simulink model "MyTransmCU_RTW"  (Simulink 10.3)
settings: Solver=ode1  StartTime=0.0  StopTime=inf  FixedStep=0.0002  RelTol=1e-3
PreLoadFcn:
  | vehicle = 'Car'; if ~length(which('cmself')), cmenv; end
  | MyTransmCU_RTW_bus
InitFcn:
  | vehicle = 'Car'; if ~length(which('cmself')), cmenv; end
  | MyTransmCU_RTW_bus
libraries: simulink x2, CarMaker4SL x1
Description:
  | CarMaker Plug-in Model Target
settings Model: Creator=IPG  LastModifiedBy=IPG  MultithreadedSim=on
settings DataIOCC: SaveFormat=Dataset  SignalLoggingSaveFormat=Dataset  ReturnWorkspaceOutputs=on
settings OptimizationCC: ExpressionDepthLimit=128  LifeSpan=auto
settings DebuggingCC: UnderspecifiedInitializationDetection=Simplified  MergeDetectMultiDrivingBlocksExec=error  FcnCallInpInsideContextMsg=error  StateNameClashWarn=none  SFUnexpectedBacktrackingDiag=error  SFNoUnconditionalDefaultTransitionDiag=error  SFExecutionAtInitializationDiag=warning  ArithmeticOperatorsInVariantConditions=error
settings HardwareCC: ProdBitPerPointer=64  ProdBitPerSizeT=64  ProdBitPerPtrDiffT=64  ProdLargestAtomicFloat=Float  ProdIntDivRoundTo=Zero  ProdEndianess=LittleEndian  ProdWordSize=64  ProdHWDeviceType=Intel->x86-64 (Windows64)
settings ModelReferenceCC: PropagateSignalLabelsOutOfModel=on
settings SFSimCC: SimUseLocalCustomCode=on  CustomCodeUndefinedFunction=FilterOut
settings RTWCC: Description=CarMaker Plug-in Model Target  SystemTargetFile=CarMaker.tlc  TemplateMakefile=CarMaker_unix-linux64.tmf  RTWUseLocalCustomCode=on
settings CodeAppCC: MaxIdLength=127  StateflowObjectComments=off
settings STFCustomTargetCC: TargetLangStandard=C99 (ISO)  CombineOutputUpdateFcns=on  MatFileLogging=on  CodeInterfacePackaging=Reusable function  GRTInterface=off  GenerateAllocFcn=on  SystemTargetFile=CarMaker.tlc
settings GRTTargetCC: TargetLangStandard=C99 (ISO)  ParMdlRefBuildCompliant=off  CompOptLevelCompliant=off  ConcurrentExecutionCompliant=off  CombineOutputUpdateFcns=on  CodeInterfacePackaging=Reusable function  CPPClassGenCompliant=off  GRTInterface=off  GenerateAllocFcn=on  UseToolchainInfoCompliant=off
settings CustomProperty: DataType=string
settings EnumStrPairs: String=Car
settings ConfigComp: CovMetricSettings=dwe  CovSaveCumulativeToWorkspaceVar=off  CovSaveSingleToWorkspaceVar=off  CovExternalEMLEnable=on

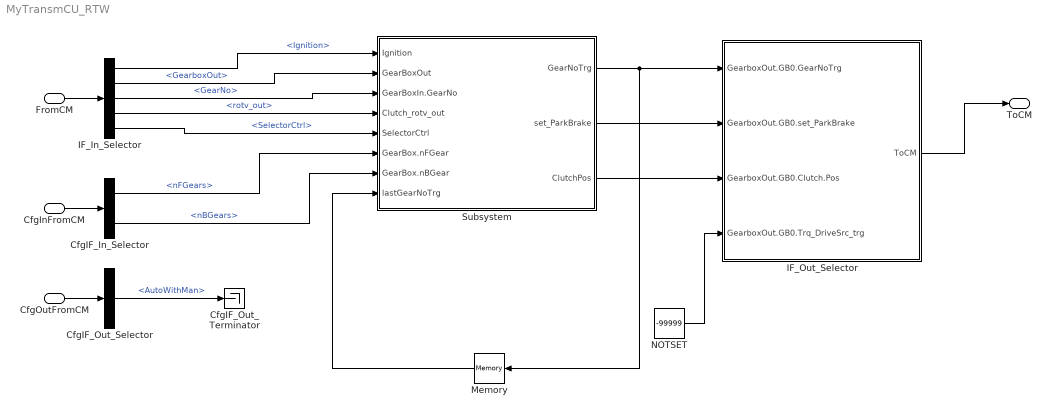
== system MyTransmCU_RTW ==
  FromCM : Inport  OutDataTypeStr=Bus: cmPTTransmCUIn
  CfgInFromCM : Inport  Port=2  OutDataTypeStr=Bus: cmPTTransmCUCfgIn
  CfgOutFromCM : Inport  Port=3  OutDataTypeStr=Bus: cmPTTransmCUCfgOut
  CfgIF_In_Selector : BusSelector  OutputSignals=Gearbox.GB0.nFGears,Gearbox.GB0.nBGears
  CfgIF_Out_Selector : BusSelector  OutputSignals=AutoWithMan
  CfgIF_Out_Terminator : Terminator
  IF_In_Selector : BusSelector  OutputSignals=Ignition,GearboxOut,GearboxIn.GB0.GearNo,GearboxIn.GB0.rotv_out,SelectorCtrl
  IF_Out_Selector : Subsystem  mask(Signal Selection){}
      mask help: Signal Selection Block
      settings: OpenFcn=cmSignalSelect('SignalSelection_CB',gcb)
  Memory : Memory
  NOTSET : Constant  Value=-99999
  Subsystem : Subsystem
  ToCM : Outport  OutDataTypeStr=Bus: cmPTTransmCUOut
  wires:
  FromCM/1 -> IF_In_Selector/1
  IF_Out_Selector/1(ToCM) -> ToCM/1
  CfgInFromCM/1 -> CfgIF_In_Selector/1
  CfgIF_In_Selector/1 -> Subsystem/6(GearBox.nFGear)  "<nFGears>"
  CfgOutFromCM/1 -> CfgIF_Out_Selector/1
  CfgIF_Out_Selector/1 -> CfgIF_Out_Terminator/1  "<AutoWithMan>"
  Memory/1 -> Subsystem/8(lastGearNoTrg)
  Subsystem/2(set_ParkBrake) -> IF_Out_Selector/2(GearboxOut.GB0.set_ParkBrake)
  IF_In_Selector/3 -> Subsystem/3(GearBoxIn.GearNo)  "<GearNo>"
  IF_In_Selector/5 -> Subsystem/5(SelectorCtrl)  "<SelectorCtrl>"
  Subsystem/3(ClutchPos) -> IF_Out_Selector/3(GearboxOut.GB0.Clutch.Pos)
  Subsystem/1(GearNoTrg) -> Memory/1, IF_Out_Selector/1(GearboxOut.GB0.GearNoTrg)
  NOTSET/1 -> IF_Out_Selector/4(GearboxOut.GB0.Trq_DriveSrc_trg)
  IF_In_Selector/4 -> Subsystem/4(Clutch_rotv_out)  "<rotv_out>"
  CfgIF_In_Selector/2 -> Subsystem/7(GearBox.nBGear)  "<nBGears>"
  IF_In_Selector/1 -> Subsystem/1(Ignition)  "<Ignition>"
  IF_In_Selector/2 -> Subsystem/2(GearBoxOut)  "<GearboxOut>"

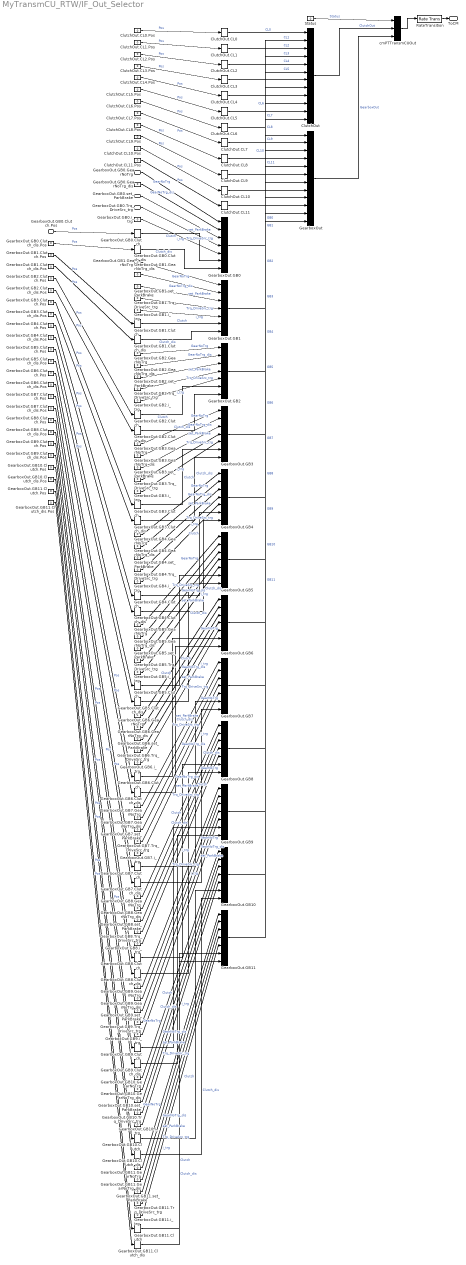
== system MyTransmCU_RTW/IF_Out_Selector ==
  GearboxOut.GB0.GearNoTrg : Inport
  GearboxOut.GB0.set_ParkBrake : Inport  Port=2
  GearboxOut.GB0.Clutch.Pos : Inport  Port=3
  GearboxOut.GB0.Trq_DriveSrc_trg : Inport  Port=4
  ClutchOut : BusCreator  Inputs=12
  ClutchOut.CL{0..11} (12 alike) : BusCreator  Inputs=1
  ClutchOut.CL0.Pos : Constant  Value=0
  ClutchOut.CL1.Pos : Constant  Value=0
  ClutchOut.CL10.Pos : Constant  Value=0
  ClutchOut.CL11.Pos : Constant  Value=0
  ClutchOut.CL2.Pos : Constant  Value=0
  ClutchOut.CL3.Pos : Constant  Value=0
  ClutchOut.CL4.Pos : Constant  Value=0
  ClutchOut.CL5.Pos : Constant  Value=0
  ClutchOut.CL6.Pos : Constant  Value=0
  ClutchOut.CL7.Pos : Constant  Value=0
  ClutchOut.CL8.Pos : Constant  Value=0
  ClutchOut.CL9.Pos : Constant  Value=0
  GearboxOut : BusCreator  Inputs=12
  GearboxOut.GB{0..11} (12 alike) : BusCreator  Inputs=7
  GearboxOut.GB0.Clutch : BusCreator  Inputs=1
  GearboxOut.GB0.Clutch_dis : BusCreator  Inputs=1
  GearboxOut.GB0.Clutch_dis.Pos : Constant  Value=0
  GearboxOut.GB0.GearNoTrg_dis : Constant  Value=0
  GearboxOut.GB0.i_trg : Constant  Value=0
  GearboxOut.GB1.Clutch : BusCreator  Inputs=1
  GearboxOut.GB1.Clutch.Pos : Constant  Value=0
  GearboxOut.GB1.Clutch_dis : BusCreator  Inputs=1
  GearboxOut.GB1.Clutch_dis.Pos : Constant  Value=0
  GearboxOut.GB1.GearNoTrg : Constant  Value=0
  GearboxOut.GB1.GearNoTrg_dis : Constant  Value=0
  GearboxOut.GB1.Trq_DriveSrc_trg : Constant  Value=0
  GearboxOut.GB1.i_trg : Constant  Value=0
  GearboxOut.GB1.set_ParkBrake : Constant  Value=0
  GearboxOut.GB10.Clutch : BusCreator  Inputs=1
  GearboxOut.GB10.Clutch.Pos : Constant  Value=0
  GearboxOut.GB10.Clutch_dis : BusCreator  Inputs=1
  GearboxOut.GB10.Clutch_dis.Pos : Constant  Value=0
  GearboxOut.GB10.GearNoTrg : Constant  Value=0
  GearboxOut.GB10.GearNoTrg_dis : Constant  Value=0
  GearboxOut.GB10.Trq_DriveSrc_trg : Constant  Value=0
  GearboxOut.GB10.i_trg : Constant  Value=0
  GearboxOut.GB10.set_ParkBrake : Constant  Value=0
  GearboxOut.GB11.Clutch : BusCreator  Inputs=1
  GearboxOut.GB11.Clutch.Pos : Constant  Value=0
  GearboxOut.GB11.Clutch_dis : BusCreator  Inputs=1
  GearboxOut.GB11.Clutch_dis.Pos : Constant  Value=0
  GearboxOut.GB11.GearNoTrg : Constant  Value=0
  GearboxOut.GB11.GearNoTrg_dis : Constant  Value=0
  GearboxOut.GB11.Trq_DriveSrc_trg : Constant  Value=0
  GearboxOut.GB11.i_trg : Constant  Value=0
  GearboxOut.GB11.set_ParkBrake : Constant  Value=0
  GearboxOut.GB2.Clutch : BusCreator  Inputs=1
  GearboxOut.GB2.Clutch.Pos : Constant  Value=0
  GearboxOut.GB2.Clutch_dis : BusCreator  Inputs=1
  GearboxOut.GB2.Clutch_dis.Pos : Constant  Value=0
  GearboxOut.GB2.GearNoTrg : Constant  Value=0
  GearboxOut.GB2.GearNoTrg_dis : Constant  Value=0
  GearboxOut.GB2.Trq_DriveSrc_trg : Constant  Value=0
  GearboxOut.GB2.i_trg : Constant  Value=0
  GearboxOut.GB2.set_ParkBrake : Constant  Value=0
  GearboxOut.GB3.Clutch : BusCreator  Inputs=1
  GearboxOut.GB3.Clutch.Pos : Constant  Value=0
  GearboxOut.GB3.Clutch_dis : BusCreator  Inputs=1
  GearboxOut.GB3.Clutch_dis.Pos : Constant  Value=0
  GearboxOut.GB3.GearNoTrg : Constant  Value=0
  GearboxOut.GB3.GearNoTrg_dis : Constant  Value=0
  GearboxOut.GB3.Trq_DriveSrc_trg : Constant  Value=0
  GearboxOut.GB3.i_trg : Constant  Value=0
  GearboxOut.GB3.set_ParkBrake : Constant  Value=0
  GearboxOut.GB4.Clutch : BusCreator  Inputs=1
  GearboxOut.GB4.Clutch.Pos : Constant  Value=0
  GearboxOut.GB4.Clutch_dis : BusCreator  Inputs=1
  GearboxOut.GB4.Clutch_dis.Pos : Constant  Value=0
  GearboxOut.GB4.GearNoTrg : Constant  Value=0
  GearboxOut.GB4.GearNoTrg_dis : Constant  Value=0
  GearboxOut.GB4.Trq_DriveSrc_trg : Constant  Value=0
  GearboxOut.GB4.i_trg : Constant  Value=0
  GearboxOut.GB4.set_ParkBrake : Constant  Value=0
  GearboxOut.GB5.Clutch : BusCreator  Inputs=1
  GearboxOut.GB5.Clutch.Pos : Constant  Value=0
  GearboxOut.GB5.Clutch_dis : BusCreator  Inputs=1
  GearboxOut.GB5.Clutch_dis.Pos : Constant  Value=0
  GearboxOut.GB5.GearNoTrg : Constant  Value=0
  GearboxOut.GB5.GearNoTrg_dis : Constant  Value=0
  GearboxOut.GB5.Trq_DriveSrc_trg : Constant  Value=0
  GearboxOut.GB5.i_trg : Constant  Value=0
  GearboxOut.GB5.set_ParkBrake : Constant  Value=0
  GearboxOut.GB6.Clutch : BusCreator  Inputs=1
  GearboxOut.GB6.Clutch.Pos : Constant  Value=0
  GearboxOut.GB6.Clutch_dis : BusCreator  Inputs=1
  GearboxOut.GB6.Clutch_dis.Pos : Constant  Value=0
  GearboxOut.GB6.GearNoTrg : Constant  Value=0
  GearboxOut.GB6.GearNoTrg_dis : Constant  Value=0
  GearboxOut.GB6.Trq_DriveSrc_trg : Constant  Value=0
  GearboxOut.GB6.i_trg : Constant  Value=0
  GearboxOut.GB6.set_ParkBrake : Constant  Value=0
  GearboxOut.GB7.Clutch : BusCreator  Inputs=1
  GearboxOut.GB7.Clutch.Pos : Constant  Value=0
  GearboxOut.GB7.Clutch_dis : BusCreator  Inputs=1
  GearboxOut.GB7.Clutch_dis.Pos : Constant  Value=0
  GearboxOut.GB7.GearNoTrg : Constant  Value=0
  GearboxOut.GB7.GearNoTrg_dis : Constant  Value=0
  GearboxOut.GB7.Trq_DriveSrc_trg : Constant  Value=0
  GearboxOut.GB7.i_trg : Constant  Value=0
  GearboxOut.GB7.set_ParkBrake : Constant  Value=0
  GearboxOut.GB8.Clutch : BusCreator  Inputs=1
  GearboxOut.GB8.Clutch.Pos : Constant  Value=0
  GearboxOut.GB8.Clutch_dis : BusCreator  Inputs=1
  GearboxOut.GB8.Clutch_dis.Pos : Constant  Value=0
  GearboxOut.GB8.GearNoTrg : Constant  Value=0
  GearboxOut.GB8.GearNoTrg_dis : Constant  Value=0
  GearboxOut.GB8.Trq_DriveSrc_trg : Constant  Value=0
  GearboxOut.GB8.i_trg : Constant  Value=0
  GearboxOut.GB8.set_ParkBrake : Constant  Value=0
  GearboxOut.GB9.Clutch : BusCreator  Inputs=1
  GearboxOut.GB9.Clutch.Pos : Constant  Value=0
  GearboxOut.GB9.Clutch_dis : BusCreator  Inputs=1
  GearboxOut.GB9.Clutch_dis.Pos : Constant  Value=0
  GearboxOut.GB9.GearNoTrg : Constant  Value=0
  GearboxOut.GB9.GearNoTrg_dis : Constant  Value=0
  GearboxOut.GB9.Trq_DriveSrc_trg : Constant  Value=0
  GearboxOut.GB9.i_trg : Constant  Value=0
  GearboxOut.GB9.set_ParkBrake : Constant  Value=0
  RateTransition : RateTransition  OutPortSampleTime=str2num(get_param(bdroot,'FixedStep'))
  Status : Constant  Value=0
  cmPTTransmCUOut : BusCreator  Inputs=3
  ToCM : Outport
  wires:
  RateTransition/1 -> ToCM/1
  cmPTTransmCUOut/1 -> RateTransition/1
  Status/1 -> cmPTTransmCUOut/1  "Status"
  ClutchOut/1 -> cmPTTransmCUOut/2  "ClutchOut"
  ClutchOut.CL0/1 -> ClutchOut/1  "CL0"
  ClutchOut.CL0.Pos/1 -> ClutchOut.CL0/1  "Pos"
  ClutchOut.CL1/1 -> ClutchOut/2  "CL1"
  ClutchOut.CL1.Pos/1 -> ClutchOut.CL1/1  "Pos"
  ClutchOut.CL2/1 -> ClutchOut/3  "CL2"
  ClutchOut.CL2.Pos/1 -> ClutchOut.CL2/1  "Pos"
  ClutchOut.CL3/1 -> ClutchOut/4  "CL3"
  ClutchOut.CL3.Pos/1 -> ClutchOut.CL3/1  "Pos"
  ClutchOut.CL4/1 -> ClutchOut/5  "CL4"
  ClutchOut.CL4.Pos/1 -> ClutchOut.CL4/1  "Pos"
  ClutchOut.CL5/1 -> ClutchOut/6  "CL5"
  ClutchOut.CL5.Pos/1 -> ClutchOut.CL5/1  "Pos"
  ClutchOut.CL6/1 -> ClutchOut/7  "CL6"
  ClutchOut.CL6.Pos/1 -> ClutchOut.CL6/1  "Pos"
  ClutchOut.CL7/1 -> ClutchOut/8  "CL7"
  ClutchOut.CL7.Pos/1 -> ClutchOut.CL7/1  "Pos"
  ClutchOut.CL8/1 -> ClutchOut/9  "CL8"
  ClutchOut.CL8.Pos/1 -> ClutchOut.CL8/1  "Pos"
  ClutchOut.CL9/1 -> ClutchOut/10  "CL9"
  ClutchOut.CL9.Pos/1 -> ClutchOut.CL9/1  "Pos"
  ClutchOut.CL10/1 -> ClutchOut/11  "CL10"
  ClutchOut.CL10.Pos/1 -> ClutchOut.CL10/1  "Pos"
  ClutchOut.CL11/1 -> ClutchOut/12  "CL11"
  ClutchOut.CL11.Pos/1 -> ClutchOut.CL11/1  "Pos"
  GearboxOut/1 -> cmPTTransmCUOut/3  "GearboxOut"
  GearboxOut.GB0/1 -> GearboxOut/1  "GB0"
  GearboxOut.GB0.GearNoTrg_dis/1 -> GearboxOut.GB0/2  "GearNoTrg_dis"
  GearboxOut.GB0.i_trg/1 -> GearboxOut.GB0/5  "i_trg"
  GearboxOut.GB0.Clutch/1 -> GearboxOut.GB0/6  "Clutch"
  GearboxOut.GB0.Clutch_dis/1 -> GearboxOut.GB0/7  "Clutch_dis"
  GearboxOut.GB0.Clutch_dis.Pos/1 -> GearboxOut.GB0.Clutch_dis/1  "Pos"
  GearboxOut.GB1/1 -> GearboxOut/2  "GB1"
  GearboxOut.GB1.GearNoTrg/1 -> GearboxOut.GB1/1  "GearNoTrg"
  GearboxOut.GB1.GearNoTrg_dis/1 -> GearboxOut.GB1/2  "GearNoTrg_dis"
  GearboxOut.GB1.set_ParkBrake/1 -> GearboxOut.GB1/3  "set_ParkBrake"
  GearboxOut.GB1.Trq_DriveSrc_trg/1 -> GearboxOut.GB1/4  "Trq_DriveSrc_trg"
  GearboxOut.GB1.i_trg/1 -> GearboxOut.GB1/5  "i_trg"
  GearboxOut.GB1.Clutch/1 -> GearboxOut.GB1/6  "Clutch"
  GearboxOut.GB1.Clutch.Pos/1 -> GearboxOut.GB1.Clutch/1  "Pos"
  GearboxOut.GB1.Clutch_dis/1 -> GearboxOut.GB1/7  "Clutch_dis"
  GearboxOut.GB1.Clutch_dis.Pos/1 -> GearboxOut.GB1.Clutch_dis/1  "Pos"
  GearboxOut.GB2/1 -> GearboxOut/3  "GB2"
  GearboxOut.GB2.GearNoTrg/1 -> GearboxOut.GB2/1  "GearNoTrg"
  GearboxOut.GB2.GearNoTrg_dis/1 -> GearboxOut.GB2/2  "GearNoTrg_dis"
  GearboxOut.GB2.set_ParkBrake/1 -> GearboxOut.GB2/3  "set_ParkBrake"
  GearboxOut.GB2.Trq_DriveSrc_trg/1 -> GearboxOut.GB2/4  "Trq_DriveSrc_trg"
  GearboxOut.GB2.i_trg/1 -> GearboxOut.GB2/5  "i_trg"
  GearboxOut.GB2.Clutch/1 -> GearboxOut.GB2/6  "Clutch"
  GearboxOut.GB2.Clutch.Pos/1 -> GearboxOut.GB2.Clutch/1  "Pos"
  GearboxOut.GB2.Clutch_dis/1 -> GearboxOut.GB2/7  "Clutch_dis"
  GearboxOut.GB2.Clutch_dis.Pos/1 -> GearboxOut.GB2.Clutch_dis/1  "Pos"
  GearboxOut.GB3/1 -> GearboxOut/4  "GB3"
  GearboxOut.GB3.GearNoTrg/1 -> GearboxOut.GB3/1  "GearNoTrg"
  GearboxOut.GB3.GearNoTrg_dis/1 -> GearboxOut.GB3/2  "GearNoTrg_dis"
  GearboxOut.GB3.set_ParkBrake/1 -> GearboxOut.GB3/3  "set_ParkBrake"
  GearboxOut.GB3.Trq_DriveSrc_trg/1 -> GearboxOut.GB3/4  "Trq_DriveSrc_trg"
  GearboxOut.GB3.i_trg/1 -> GearboxOut.GB3/5  "i_trg"
  GearboxOut.GB3.Clutch/1 -> GearboxOut.GB3/6  "Clutch"
  GearboxOut.GB3.Clutch.Pos/1 -> GearboxOut.GB3.Clutch/1  "Pos"
  GearboxOut.GB3.Clutch_dis/1 -> GearboxOut.GB3/7  "Clutch_dis"
  GearboxOut.GB3.Clutch_dis.Pos/1 -> GearboxOut.GB3.Clutch_dis/1  "Pos"
  GearboxOut.GB4/1 -> GearboxOut/5  "GB4"
  GearboxOut.GB4.GearNoTrg/1 -> GearboxOut.GB4/1  "GearNoTrg"
  GearboxOut.GB4.GearNoTrg_dis/1 -> GearboxOut.GB4/2  "GearNoTrg_dis"
  GearboxOut.GB4.set_ParkBrake/1 -> GearboxOut.GB4/3  "set_ParkBrake"
  GearboxOut.GB4.Trq_DriveSrc_trg/1 -> GearboxOut.GB4/4  "Trq_DriveSrc_trg"
  GearboxOut.GB4.i_trg/1 -> GearboxOut.GB4/5  "i_trg"
  GearboxOut.GB4.Clutch/1 -> GearboxOut.GB4/6  "Clutch"
  GearboxOut.GB4.Clutch.Pos/1 -> GearboxOut.GB4.Clutch/1  "Pos"
  GearboxOut.GB4.Clutch_dis/1 -> GearboxOut.GB4/7  "Clutch_dis"
  GearboxOut.GB4.Clutch_dis.Pos/1 -> GearboxOut.GB4.Clutch_dis/1  "Pos"
  GearboxOut.GB5/1 -> GearboxOut/6  "GB5"
  GearboxOut.GB5.GearNoTrg/1 -> GearboxOut.GB5/1  "GearNoTrg"
  GearboxOut.GB5.GearNoTrg_dis/1 -> GearboxOut.GB5/2  "GearNoTrg_dis"
  GearboxOut.GB5.set_ParkBrake/1 -> GearboxOut.GB5/3  "set_ParkBrake"
  GearboxOut.GB5.Trq_DriveSrc_trg/1 -> GearboxOut.GB5/4  "Trq_DriveSrc_trg"
  GearboxOut.GB5.i_trg/1 -> GearboxOut.GB5/5  "i_trg"
  GearboxOut.GB5.Clutch/1 -> GearboxOut.GB5/6  "Clutch"
  GearboxOut.GB5.Clutch.Pos/1 -> GearboxOut.GB5.Clutch/1  "Pos"
  GearboxOut.GB5.Clutch_dis/1 -> GearboxOut.GB5/7  "Clutch_dis"
  GearboxOut.GB5.Clutch_dis.Pos/1 -> GearboxOut.GB5.Clutch_dis/1  "Pos"
  GearboxOut.GB6/1 -> GearboxOut/7  "GB6"
  GearboxOut.GB6.GearNoTrg/1 -> GearboxOut.GB6/1  "GearNoTrg"
  GearboxOut.GB6.GearNoTrg_dis/1 -> GearboxOut.GB6/2  "GearNoTrg_dis"
  GearboxOut.GB6.set_ParkBrake/1 -> GearboxOut.GB6/3  "set_ParkBrake"
  GearboxOut.GB6.Trq_DriveSrc_trg/1 -> GearboxOut.GB6/4  "Trq_DriveSrc_trg"
  GearboxOut.GB6.i_trg/1 -> GearboxOut.GB6/5  "i_trg"
  GearboxOut.GB6.Clutch/1 -> GearboxOut.GB6/6  "Clutch"
  GearboxOut.GB6.Clutch.Pos/1 -> GearboxOut.GB6.Clutch/1  "Pos"
  GearboxOut.GB6.Clutch_dis/1 -> GearboxOut.GB6/7  "Clutch_dis"
  GearboxOut.GB6.Clutch_dis.Pos/1 -> GearboxOut.GB6.Clutch_dis/1  "Pos"
  GearboxOut.GB7/1 -> GearboxOut/8  "GB7"
  GearboxOut.GB7.GearNoTrg/1 -> GearboxOut.GB7/1  "GearNoTrg"
  GearboxOut.GB7.GearNoTrg_dis/1 -> GearboxOut.GB7/2  "GearNoTrg_dis"
  GearboxOut.GB7.set_ParkBrake/1 -> GearboxOut.GB7/3  "set_ParkBrake"
  GearboxOut.GB7.Trq_DriveSrc_trg/1 -> GearboxOut.GB7/4  "Trq_DriveSrc_trg"
  GearboxOut.GB7.i_trg/1 -> GearboxOut.GB7/5  "i_trg"
  GearboxOut.GB7.Clutch/1 -> GearboxOut.GB7/6  "Clutch"
  GearboxOut.GB7.Clutch.Pos/1 -> GearboxOut.GB7.Clutch/1  "Pos"
  GearboxOut.GB7.Clutch_dis/1 -> GearboxOut.GB7/7  "Clutch_dis"
  GearboxOut.GB7.Clutch_dis.Pos/1 -> GearboxOut.GB7.Clutch_dis/1  "Pos"
  GearboxOut.GB8/1 -> GearboxOut/9  "GB8"
  GearboxOut.GB8.GearNoTrg/1 -> GearboxOut.GB8/1  "GearNoTrg"
  GearboxOut.GB8.GearNoTrg_dis/1 -> GearboxOut.GB8/2  "GearNoTrg_dis"
  GearboxOut.GB8.set_ParkBrake/1 -> GearboxOut.GB8/3  "set_ParkBrake"
  GearboxOut.GB8.Trq_DriveSrc_trg/1 -> GearboxOut.GB8/4  "Trq_DriveSrc_trg"
  GearboxOut.GB8.i_trg/1 -> GearboxOut.GB8/5  "i_trg"
  GearboxOut.GB8.Clutch/1 -> GearboxOut.GB8/6  "Clutch"
  GearboxOut.GB8.Clutch.Pos/1 -> GearboxOut.GB8.Clutch/1  "Pos"
  GearboxOut.GB8.Clutch_dis/1 -> GearboxOut.GB8/7  "Clutch_dis"
  GearboxOut.GB8.Clutch_dis.Pos/1 -> GearboxOut.GB8.Clutch_dis/1  "Pos"
  GearboxOut.GB9/1 -> GearboxOut/10  "GB9"
  GearboxOut.GB9.GearNoTrg/1 -> GearboxOut.GB9/1  "GearNoTrg"
  GearboxOut.GB9.GearNoTrg_dis/1 -> GearboxOut.GB9/2  "GearNoTrg_dis"
  GearboxOut.GB9.set_ParkBrake/1 -> GearboxOut.GB9/3  "set_ParkBrake"
  GearboxOut.GB9.Trq_DriveSrc_trg/1 -> GearboxOut.GB9/4  "Trq_DriveSrc_trg"
  GearboxOut.GB9.i_trg/1 -> GearboxOut.GB9/5  "i_trg"
  GearboxOut.GB9.Clutch/1 -> GearboxOut.GB9/6  "Clutch"
  GearboxOut.GB9.Clutch.Pos/1 -> GearboxOut.GB9.Clutch/1  "Pos"
  GearboxOut.GB9.Clutch_dis/1 -> GearboxOut.GB9/7  "Clutch_dis"
  GearboxOut.GB9.Clutch_dis.Pos/1 -> GearboxOut.GB9.Clutch_dis/1  "Pos"
  GearboxOut.GB10/1 -> GearboxOut/11  "GB10"
  GearboxOut.GB10.GearNoTrg/1 -> GearboxOut.GB10/1  "GearNoTrg"
  GearboxOut.GB10.GearNoTrg_dis/1 -> GearboxOut.GB10/2  "GearNoTrg_dis"
  GearboxOut.GB10.set_ParkBrake/1 -> GearboxOut.GB10/3  "set_ParkBrake"
  GearboxOut.GB10.Trq_DriveSrc_trg/1 -> GearboxOut.GB10/4  "Trq_DriveSrc_trg"
  GearboxOut.GB10.i_trg/1 -> GearboxOut.GB10/5  "i_trg"
  GearboxOut.GB10.Clutch/1 -> GearboxOut.GB10/6  "Clutch"
  GearboxOut.GB10.Clutch.Pos/1 -> GearboxOut.GB10.Clutch/1  "Pos"
  GearboxOut.GB10.Clutch_dis/1 -> GearboxOut.GB10/7  "Clutch_dis"
  GearboxOut.GB10.Clutch_dis.Pos/1 -> GearboxOut.GB10.Clutch_dis/1  "Pos"
  GearboxOut.GB11/1 -> GearboxOut/12  "GB11"
  GearboxOut.GB11.GearNoTrg/1 -> GearboxOut.GB11/1  "GearNoTrg"
  GearboxOut.GB11.GearNoTrg_dis/1 -> GearboxOut.GB11/2  "GearNoTrg_dis"
  GearboxOut.GB11.set_ParkBrake/1 -> GearboxOut.GB11/3  "set_ParkBrake"
  GearboxOut.GB11.Trq_DriveSrc_trg/1 -> GearboxOut.GB11/4  "Trq_DriveSrc_trg"
  GearboxOut.GB11.i_trg/1 -> GearboxOut.GB11/5  "i_trg"
  GearboxOut.GB11.Clutch/1 -> GearboxOut.GB11/6  "Clutch"
  GearboxOut.GB11.Clutch.Pos/1 -> GearboxOut.GB11.Clutch/1  "Pos"
  GearboxOut.GB11.Clutch_dis/1 -> GearboxOut.GB11/7  "Clutch_dis"
  GearboxOut.GB11.Clutch_dis.Pos/1 -> GearboxOut.GB11.Clutch_dis/1  "Pos"
  GearboxOut.GB0.GearNoTrg/1 -> GearboxOut.GB0/1  "GearNoTrg"
  GearboxOut.GB0.set_ParkBrake/1 -> GearboxOut.GB0/3  "set_ParkBrake"
  GearboxOut.GB0.Clutch.Pos/1 -> GearboxOut.GB0.Clutch/1  "Pos"
  GearboxOut.GB0.Trq_DriveSrc_trg/1 -> GearboxOut.GB0/4  "Trq_DriveSrc_trg"

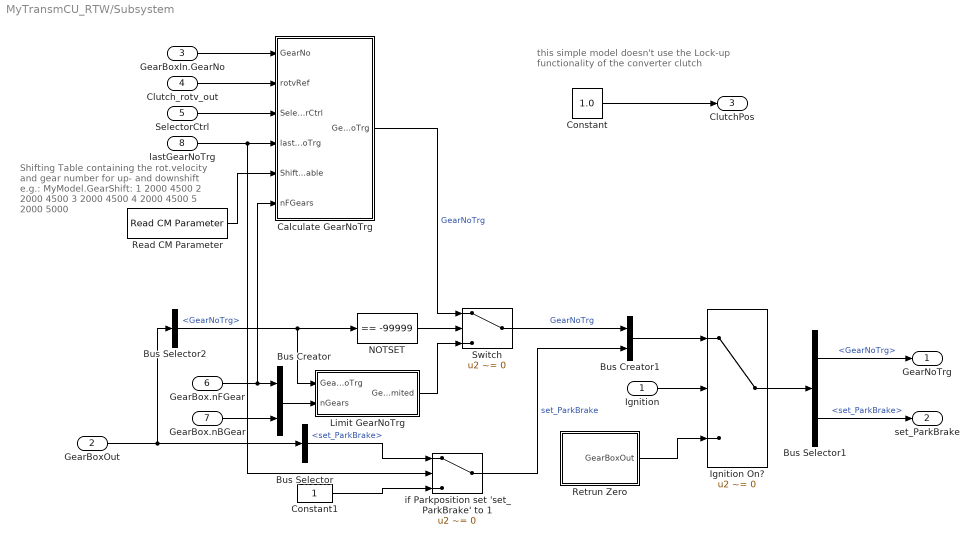
== system MyTransmCU_RTW/Subsystem ==
  note: Shifting Table containing the rot.velocity
      | and gear number for up- and downshift
      | e.g.:
      | MyModel.GearShift:
      |     1    2000    4500
      |     2    2000    4500
      |     3    2000    4500
      |     4    2000    4500
      |     5    2000    5000
  note: this simple model doesn't use the
      | Lock-up functionality of the converter clutch
  Ignition : Inport
  GearBoxOut : Inport  Port=2
  GearBoxIn.GearNo : Inport  Port=3
  Clutch_rotv_out : Inport  Port=4
  SelectorCtrl : Inport  Port=5
  GearBox.nFGear : Inport  Port=6
  GearBox.nBGear : Inport  Port=7
  lastGearNoTrg : Inport  Port=8
  Bus Creator : BusCreator  Inputs=2
  Bus Creator1 : BusCreator  Inputs=2
  Bus Selector : BusSelector  OutputSignals=GB0.set_ParkBrake
  Bus Selector1 : BusSelector  OutputSignals=GearNoTrg,set_ParkBrake
  Bus Selector2 : BusSelector  OutputSignals=GB0.GearNoTrg
  Calculate GearNoTrg : Subsystem  TreatAsAtomicUnit=on
  Constant : Constant  Value=1.0
  Constant1 : Constant
  Ignition On? : Switch  Criteria=u2 ~= 0
  Limit GearNoTrg : Subsystem
  NOTSET : simulink/Logic and Bit Operations/Compare To Constant  relop===  const=-99999  OutDataTypeStr=uint8
  Read CM Parameter : CarMaker4SL/Read CM Parameter  xfile=Vehicle  xkey=MyModel.GearShift  xnout=80  xdefaults=0  xmuxed=on  xstime=Continuous
      settings: SourceProductName=CarMaker4SL
  Retrun Zero : Subsystem  TreatAsAtomicUnit=on
  Switch : Switch  Criteria=u2 ~= 0
  if Parkposition set 'set_ParkBrake' to 1 : Switch  Criteria=u2 ~= 0
  GearNoTrg : Outport  VectorParamsAs1DForOutWhenUnconnected=off
  set_ParkBrake : Outport  Port=2  VectorParamsAs1DForOutWhenUnconnected=off
  ClutchPos : Outport  Port=3  VectorParamsAs1DForOutWhenUnconnected=off
  wires:
  Constant1/1 -> if Parkposition set 'set_ParkBrake' to 1/3
  Bus Selector/1 -> if Parkposition set 'set_ParkBrake' to 1/1  "<set_ParkBrake>"
  if Parkposition set 'set_ParkBrake' to 1/1 -> Bus Creator1/2  "set_ParkBrake"
  lastGearNoTrg/1 -> if Parkposition set 'set_ParkBrake' to 1/2, Calculate GearNoTrg/4(lastGearNoTrg)
  Limit GearNoTrg/1(GearNoTrg_limited) -> Switch/3
  Calculate GearNoTrg/1(GearNoTrg) -> Switch/1  "GearNoTrg"
  Switch/1 -> Bus Creator1/1  "GearNoTrg"
  Bus Creator1/1 -> Ignition On?/1
  Retrun Zero/1(GearBoxOut) -> Ignition On?/3
  Read CM Parameter/1 -> Calculate GearNoTrg/5(ShiftingTable)
  SelectorCtrl/1 -> Calculate GearNoTrg/3(SelectorCtrl)
  Clutch_rotv_out/1 -> Calculate GearNoTrg/2(rotvRef)
  Ignition/1 -> Ignition On?/2
  Bus Creator/1 -> Limit GearNoTrg/2(nGears)
  Bus Selector2/1 -> Limit GearNoTrg/1(GearNoTrg), NOTSET/1  "<GearNoTrg>"
  NOTSET/1 -> Switch/2
  Constant/1 -> ClutchPos/1
  Bus Selector1/2 -> set_ParkBrake/1  "<set_ParkBrake>"
  Bus Selector1/1 -> GearNoTrg/1  "<GearNoTrg>"
  Ignition On?/1 -> Bus Selector1/1
  GearBoxIn.GearNo/1 -> Calculate GearNoTrg/1(GearNo)
  GearBox.nBGear/1 -> Bus Creator/2
  GearBox.nFGear/1 -> Calculate GearNoTrg/6(nFGears), Bus Creator/1
  GearBoxOut/1 -> Bus Selector2/1, Bus Selector/1

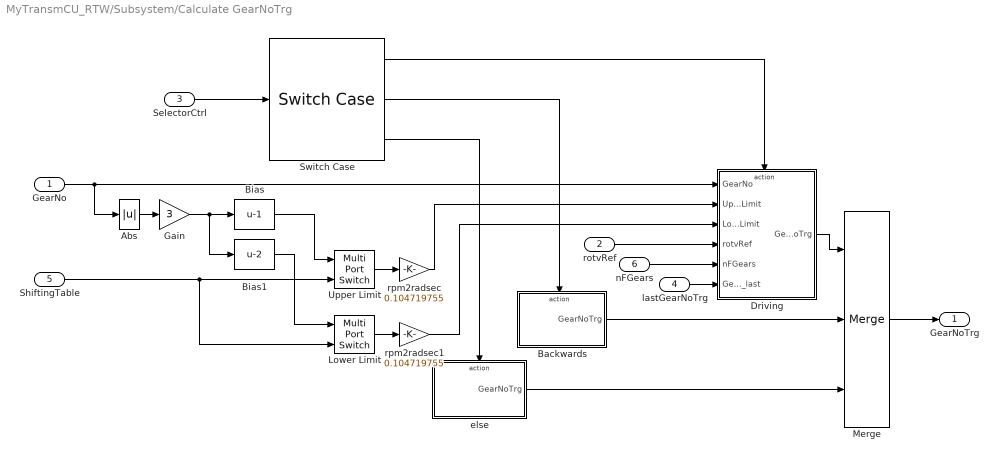
== system MyTransmCU_RTW/Subsystem/Calculate GearNoTrg ==
  GearNo : Inport
  rotvRef : Inport  Port=2
  SelectorCtrl : Inport  Port=3
  lastGearNoTrg : Inport  Port=4
  ShiftingTable : Inport  Port=5
  nFGears : Inport  Port=6
  Abs : Abs
  Backwards : Subsystem  TreatAsAtomicUnit=on
  Bias : Bias  Bias=-1
  Bias1 : Bias  Bias=-2
  Driving : Subsystem  TreatAsAtomicUnit=on
  Gain : Gain  Gain=3
  Lower Limit : MultiPortSwitch  DataPortOrder=Zero-based contiguous  Inputs=1  zeroidx=on
  Merge : Merge  Inputs=3
  Switch Case : SwitchCase  CaseConditions={1,-1}
  Upper Limit : MultiPortSwitch  DataPortOrder=Zero-based contiguous  Inputs=1  zeroidx=on
  else : Subsystem  TreatAsAtomicUnit=on
  rpm2radsec : Gain  Gain=0.104719755
  rpm2radsec1 : Gain  Gain=0.104719755
  GearNoTrg : Outport  VectorParamsAs1DForOutWhenUnconnected=off
  wires:
  lastGearNoTrg/1 -> Driving/6(GearNoTrg_last)
  nFGears/1 -> Driving/5(nFGears)
  rpm2radsec1/1 -> Driving/3(Lower Limit)
  rpm2radsec/1 -> Driving/2(Upper Limit)
  rotvRef/1 -> Driving/4(rotvRef)
  Abs/1 -> Gain/1
  Switch Case/3 -> else/Action
  Switch Case/2 -> Backwards/Action
  Merge/1 -> GearNoTrg/1
  else/1(GearNoTrg) -> Merge/3
  Backwards/1(GearNoTrg) -> Merge/2
  Driving/1(GearNoTrg) -> Merge/1
  Switch Case/1 -> Driving/Action
  SelectorCtrl/1 -> Switch Case/1
  Lower Limit/1 -> rpm2radsec1/1
  GearNo/1 -> Driving/1(GearNo), Abs/1
  Bias1/1 -> Lower Limit/1
  Gain/1 -> Bias1/1, Bias/1
  ShiftingTable/1 -> Lower Limit/2, Upper Limit/2
  Bias/1 -> Upper Limit/1
  Upper Limit/1 -> rpm2radsec/1

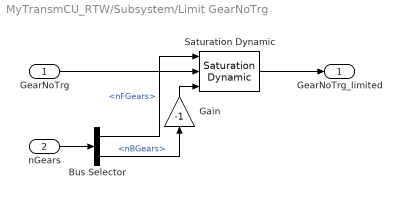
== system MyTransmCU_RTW/Subsystem/Limit GearNoTrg ==
  GearNoTrg : Inport
  nGears : Inport  Port=2
  Bus Selector : BusSelector  OutputSignals=nFGears,nBGears
  Gain : Gain  Gain=-1
  Saturation Dynamic : simulink/Discontinuities/Saturation Dynamic  OutMin=[]  OutMax=[]  OutDataTypeStr=Inherit: Same as second input  OutDataType=sfix(16)  OutScaling=2^-10  DoSatur=off
  GearNoTrg_limited : Outport  VectorParamsAs1DForOutWhenUnconnected=off
  wires:
  nGears/1 -> Bus Selector/1
  Saturation Dynamic/1 -> GearNoTrg_limited/1
  Gain/1 -> Saturation Dynamic/3
  Bus Selector/2 -> Gain/1  "<nBGears>"
  Bus Selector/1 -> Saturation Dynamic/1  "<nFGears>"
  GearNoTrg/1 -> Saturation Dynamic/2

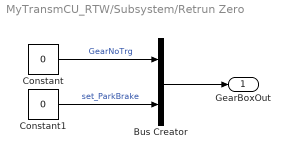
== system MyTransmCU_RTW/Subsystem/Retrun Zero ==
  Bus Creator : BusCreator  Inputs=2
  Constant : Constant  Value=0
  Constant1 : Constant  Value=0
  GearBoxOut : Outport  VectorParamsAs1DForOutWhenUnconnected=off
  wires:
  Bus Creator/1 -> GearBoxOut/1
  Constant1/1 -> Bus Creator/2  "set_ParkBrake"
  Constant/1 -> Bus Creator/1  "GearNoTrg"

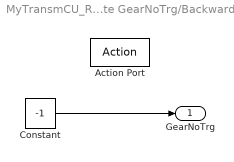
== system MyTransmCU_RTW/Subsystem/Calculate GearNoTrg/Backwards ==
  Action Port : ActionPort
  Constant : Constant  Value=-1
  GearNoTrg : Outport  InitialOutput=-1  VectorParamsAs1DForOutWhenUnconnected=off
  wires:
  Constant/1 -> GearNoTrg/1

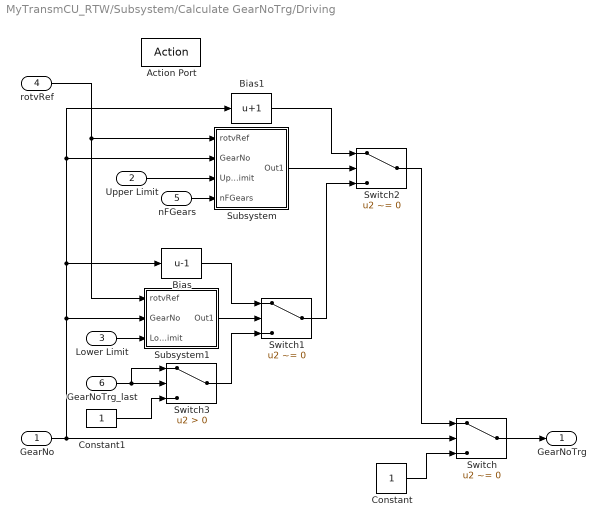
== system MyTransmCU_RTW/Subsystem/Calculate GearNoTrg/Driving ==
  GearNo : Inport
  Upper Limit : Inport  Port=2
  Lower Limit : Inport  Port=3
  rotvRef : Inport  Port=4
  nFGears : Inport  Port=5
  GearNoTrg_last : Inport  Port=6
  Action Port : ActionPort
  Bias : Bias  Bias=-1
  Bias1 : Bias  Bias=1
  Constant : Constant
  Constant1 : Constant
  Subsystem : Subsystem
  Subsystem1 : Subsystem
  Switch : Switch  Criteria=u2 ~= 0
  Switch1 : Switch  Criteria=u2 ~= 0
  Switch2 : Switch  Criteria=u2 ~= 0
  Switch3 : Switch  Criteria=u2 > Threshold
  GearNoTrg : Outport  VectorParamsAs1DForOutWhenUnconnected=off
  wires:
  Constant1/1 -> Switch3/3
  GearNoTrg_last/1 -> Switch3/1, Switch3/2
  Switch3/1 -> Switch1/3
  Lower Limit/1 -> Subsystem1/3(Lower Limit)
  Subsystem1/1(Out1) -> Switch1/2
  nFGears/1 -> Subsystem/4(nFGears)
  Upper Limit/1 -> Subsystem/3(Upper Limit)
  Subsystem/1(Out1) -> Switch2/2
  Bias1/1 -> Switch2/1
  Bias/1 -> Switch1/1
  Switch1/1 -> Switch2/3
  Switch2/1 -> Switch/1
  rotvRef/1 -> Subsystem1/1(rotvRef), Subsystem/1(rotvRef)
  Switch/1 -> GearNoTrg/1
  Constant/1 -> Switch/3
  GearNo/1 -> Switch/2, Subsystem1/2(GearNo), Subsystem/2(GearNo), Bias1/1, Bias/1

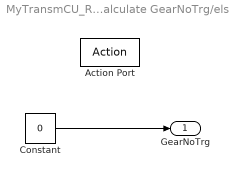
== system MyTransmCU_RTW/Subsystem/Calculate GearNoTrg/else ==
  Action Port : ActionPort
  Constant : Constant  Value=0
  GearNoTrg : Outport  InitialOutput=0  VectorParamsAs1DForOutWhenUnconnected=off
  wires:
  Constant/1 -> GearNoTrg/1

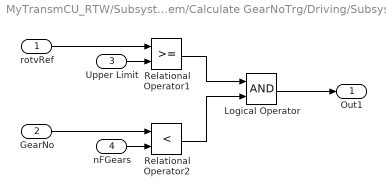
== system MyTransmCU_RTW/Subsystem/Calculate GearNoTrg/Driving/Subsystem ==
  rotvRef : Inport
  GearNo : Inport  Port=2
  Upper Limit : Inport  Port=3
  nFGears : Inport  Port=4
  Logical Operator : Logic  AllPortsSameDT=off  OutDataTypeStr=boolean
  Relational Operator1 : RelationalOperator  OutDataTypeStr=boolean  RndMeth=Nearest
  Relational Operator2 : RelationalOperator  Operator=<  OutDataTypeStr=boolean  RndMeth=Nearest
  Out1 : Outport  VectorParamsAs1DForOutWhenUnconnected=off
  wires:
  Relational Operator2/1 -> Logical Operator/2
  nFGears/1 -> Relational Operator2/2
  GearNo/1 -> Relational Operator2/1
  Logical Operator/1 -> Out1/1
  Relational Operator1/1 -> Logical Operator/1
  Upper Limit/1 -> Relational Operator1/2
  rotvRef/1 -> Relational Operator1/1

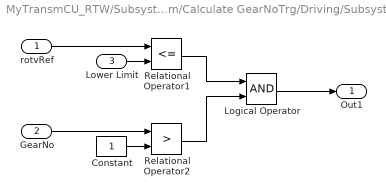
== system MyTransmCU_RTW/Subsystem/Calculate GearNoTrg/Driving/Subsystem1 ==
  rotvRef : Inport
  GearNo : Inport  Port=2
  Lower Limit : Inport  Port=3
  Constant : Constant
  Logical Operator : Logic  AllPortsSameDT=off  OutDataTypeStr=boolean
  Relational Operator1 : RelationalOperator  Operator=<=  OutDataTypeStr=boolean  RndMeth=Nearest
  Relational Operator2 : RelationalOperator  Operator=>  OutDataTypeStr=boolean  RndMeth=Nearest
  Out1 : Outport  VectorParamsAs1DForOutWhenUnconnected=off
  wires:
  Relational Operator2/1 -> Logical Operator/2
  Constant/1 -> Relational Operator2/2
  GearNo/1 -> Relational Operator2/1
  Logical Operator/1 -> Out1/1
  Relational Operator1/1 -> Logical Operator/1
  Lower Limit/1 -> Relational Operator1/2
  rotvRef/1 -> Relational Operator1/1
